simulink model "DoubleWishbone"  (Simulink 9.3)
settings: Solver=ode45  StartTime=0.0  StopTime=0.066  RelTol=1e-3  EnableMultiTasking=on
values from neighbouring files (symbols this model uses):
  s = solve(eqn,x)    [solver.m]
undefined symbols (not defined in the file): x
libraries: mblibv1 x47
settings Model: Creator=tdenery  LastModifiedBy=nicwiggins
settings DataIOCC: LimitDataPoints=on
settings OptimizationCC: InitFltsAndDblsToZero=on
settings DebuggingCC: SaveWithParameterizedLinksMsg=none  SignalResolutionControl=TryResolveAllWithWarning  MultiTaskDSMMsg=warning  MultiTaskCondExecSysMsg=none
settings HardwareCC: TargetBitPerLong=64  TargetBitPerPointer=64  TargetBitPerSizeT=64  TargetBitPerPtrDiffT=64  TargetLongLongMode=on  TargetIntDivRoundTo=Zero  TargetEndianess=LittleEndian  TargetWordSize=64  TargetHWDeviceType=MATLAB Host  ProdEqTarget=off
settings SFSimCC: SimUseLocalCustomCode=on
settings RTWCC: RTWUseLocalCustomCode=on
settings GRTTargetCC: TargetFcnLib=ansi_tfl_tmw.mat
settings ConfigComp: CovExternalEMLEnable=on

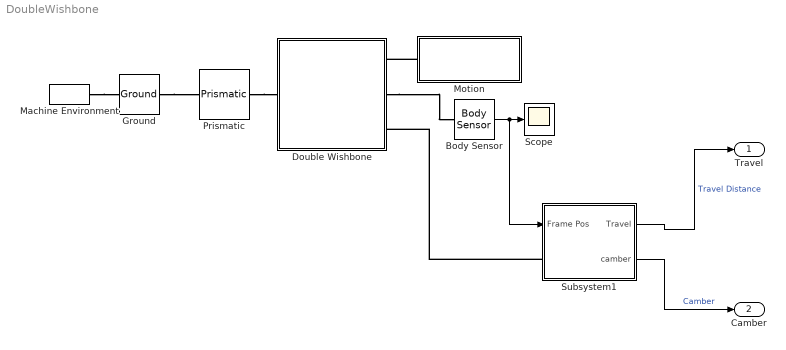
== system DoubleWishbone ==
  Body Sensor : mblibv1/Sensors &  Actuators/Body Sensor  UpdateFromCAD=off  PhysicalDomain=Mechanical  PortType=blob  Muxed=on  Pose=off  Angle=on  AngleUnits=deg  ArcVelocity=off  ArcVelocityUnits=deg/s  ArcAcceleration=off  ArcAccelerationUnits=deg/s^2  CoordPosition=on  CoordPositionUnits=m  Velocity=off  VelocityUnits=m/s  Acceleration=off  AccelerationUnits=m/s^2  Quaternion=on  QuaternionDT=off  QuaternionDDT=off  QuaternionUnits=off  OutputVector=[ 3 ]  ActiveIO=on  Width=3  DialogClass=MechanicalSensorBlock  ReferenceFrame=Absolute (World)
      settings: SourceProductName=Simscape Multibody  SourceProductBaseCode=MS
  Double Wishbone : Subsystem  mask(Double Wishbone Suspension){LU=x(1), UFPt=x(2:4), UBPt=x(5:7), LL=x(8), LFPt=x(9:11), LBPt=x(12:14), LC=x(15), k=300, b=20, Fps=20000}
      mask prompts: LU "Upper Arm Length (in)"; UFPt "Upper Arm Front Connection Point [x y z] (in)"; UBPt "Upper Arm Back Connection Point [x y z] (in)"; LL "Lower Arm Length (in)"; LFPt "Lower Arm Front Connection Point [x y z] (in)"; LBPt "Lower Arm Back Connection Point [x y z] (in)"; LC "Connecting Ling Length (in)"; k "Shock Spring Constant (lbf/in)"; b "Shock Damping Constant (lbf-s/in)"; Fps "Shock Pre-Set Force (lbf)"
      mask init:
      | UPV = UBPt - UFPt;
      | UBase = sqrt(UPV(1)^2+UPV(2)^2+UPV(3)^2);
      | ULink = sqrt(LU*LU + UBase*UBase/4);
      | LPV = LBPt - LFPt;
      | LBase = sqrt(LPV(1)^2+LPV(2)^2+LPV(3)^2);
      | LLink = sqrt(LL*LL + LBase*LBase/4);
  Ground : mblibv1/Bodies/Ground  UpdateFromCAD=off  LeftPortType=env  RightPortType=workingframe  PhysicalDomain=Mechanical  DialogClass=GroundBlock  CoordPosition=[0 0 0]  CoordPositionUnits=m  StateVectorMgrId=-1  MachineId=[0 0]  ShowEnvPort=on  ParameterChecksum=[0 0 0 0]  TopologyChecksum=[0 0 0 0]
      settings: SourceProductName=Simscape Multibody  SourceProductBaseCode=MS
  Machine Environment : mblibv1/Bodies/Machine Environment  Tag=Factory ground  PortType=env  PhysicalDomain=Mechanical  DialogTemplateClass=MECH.MachineEnvironment  SyncWhenCopied=off  Gravity=[0 -9.81 0]  GravityUnits=m/s^2  GravityAsSignal=off  Dimensionality=Auto-detect  AnalysisType=Forward dynamics  LinearAssemblyTolerance=1e-3  LinearAssemblyToleranceUnits=m  AngularAssemblyTolerance=1e-3  AngularAssemblyToleranceUnits=rad  ConstraintSolverType=Stabilizing  ConstraintRelTolerance=1e-4  ConstraintAbsTolerance=1e-4  UseRobustSingularityHandling=off  RedundancyAnalysisToleranceType=Automatically select tolerance  RedundancyAnalysisTolerance=1e-14  StatePerturbationType=Fixed  PerturbationSize=1e-5  VisualizeMachine=on  BodyVisualizationType=Use model default body geometries  BodyColorSelMode=Use model default  DefaultBodyColor=[1 0 0]
      settings: SourceProductName=Simscape Multibody  SourceProductBaseCode=MS
  Motion : Subsystem  mask{dhole=0.2, dtravel=30, speed=10}
      mask prompts: dhole "Pot Hole Depth (m)"; dtravel "Travel Distance to Hole (m)"; speed "Vehicle Speed (m/s)"
  Prismatic : mblibv1/Joints/Prismatic  LConnTagsString=__newl0  RConnTagsString=__newr0  UpdateFromCAD=off  NumSAPorts=0  CutJoint=off  MarkAsCut=off  Primitives=prismatic  PrimitiveProps=P1$WORLD$[0 1 0]$prismatic  DialogClass=JointBlock  P1Axis=[0 1 0]
      settings: SourceProductName=Simscape Multibody  SourceProductBaseCode=MS
  Scope : Scope
  Subsystem1 : Subsystem
  Travel : Outport
  Camber : Outport  Port=2
  wires:
  Body Sensor/1 -> Scope/1, Subsystem1/1(Frame Pos)
  Subsystem1/1(Travel) -> Travel/1  "Travel Distance"
  Subsystem1/2(camber) -> Camber/1  "Camber"
  connections:
  Machine Environment/RConn1 -- Ground/LConn1
  Ground/RConn1 -- Prismatic/LConn1
  Prismatic/RConn1 -- Double Wishbone/LConn1
  Motion/LConn1 -- Double Wishbone/RConn1
  Double Wishbone/RConn2 -- Body Sensor/LConn1
  Subsystem1/LConn1 -- Double Wishbone/RConn3

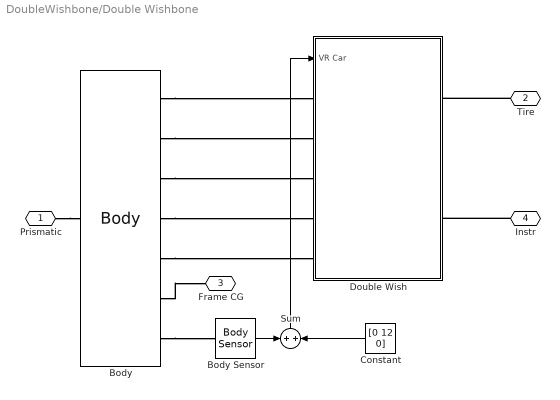
== system DoubleWishbone/Double Wishbone ==
  Body : mblibv1/Bodies/Body  LConnTagsString=CS1  RConnTagsString=CS2|CS3|CS4|CS5|CS6|CS7|CS8  UpdateFromCAD=off  DialogClass=MechanicalBodyBlock  Mass=1000  MassUnits=lbm  InertiaUnits=lbm*in^2  Inertia=eye(3)  Shape=Cylinder  ShapeDims=[1 1]  ShapeUnits=m  ShapeUse=false  Density=1  DensityUnits=kg/m^3  DensityUse=false  GraphicsMode=MACHINE_DEFAULT  BodyColorSelMode=MACHINE_DEFAULT  BodyColor=[1;0;0]  AttachedToCS=CG  CG=Left$CG$[0 0 0]$CS1$CS1$in$[0 0 0]$Euler X-Y-Z$deg$CS1$false  WorkingFrames=Left$CS1$[0 0 0]$ADJOINING$ADJOINING$in$[0 0 0]$Euler X-Y-Z$deg$ADJOINING$true#Right$CS2$UFPt$CG$CG$in$[0 0 0]$Euler X-Y-Z$deg$CG$true#Right$CS3$UBPt$CG$CG$in$[0 0 0]$Euler X-Y-Z$deg$CG$true#Right$CS4$LFPt$CG$CG$in$[0 0 0]$Euler X-Y-Z$deg$CG$true#Right$CS5$LBPt$CG$CG$in$[0 0 0]$Euler X-Y-Z$deg$CG$true#Right$CS6$[0 0 0]$ADJOINING$ADJOINING$in$[0 0 0]$Euler X-Y-Z$deg$ADJOINING$true#Right$CS7$[0 0 0]$CG$CG$in$[0 0 0]$Euler X-Y-Z$deg$WORLD$true#Right$CS8$[0 0 0]$CG$CG$m$[0 0 0]$Euler X-Y-Z$deg$CG$true  CGPos=[0 0 0]  CGRot=[0 0 0]  CS0Pos=[]  CS0Rot=[]  CS1Pos=[0 0 0]  CS1Rot=[0 0 0]  CS2Pos=UFPt  CS2Rot=[0 0 0]  CS3Pos=UBPt  CS3Rot=[0 0 0]  CS4Pos=LFPt  CS4Rot=[0 0 0]  CS5Pos=LBPt  CS5Rot=[0 0 0]  CS6Pos=[0 0 0]  CS6Rot=[0 0 0]  CS7Pos=[0 0 0]  CS7Rot=[0 0 0]  CS8Pos=[0 0 0]  CS8Rot=[0 0 0]  CS9Pos=[]  CS9Rot=[]  CS10Pos=[]  CS10Rot=[]  CS11Pos=[]  CS11Rot=[]  CS12Pos=[]  CS12Rot=[]  CS13Pos=[]  CS13Rot=[]  CS14Pos=[]  CS14Rot=[]  CS15Pos=[]  CS15Rot=[]  CS16Pos=[]  CS16Rot=[]  CS17Pos=[]  CS17Rot=[]  CS18Pos=[]  CS18Rot=[]  CS19Pos=[]  CS19Rot=[]  CS20Pos=[]  CS20Rot=[]
      settings: SourceProductName=Simscape Multibody  SourceProductBaseCode=MS
  Body Sensor : mblibv1/Sensors &  Actuators/Body Sensor  UpdateFromCAD=off  PhysicalDomain=Mechanical  PortType=blob  Muxed=on  Pose=off  Angle=on  AngleUnits=deg  ArcVelocity=off  ArcVelocityUnits=deg/s  ArcAcceleration=off  ArcAccelerationUnits=deg/s^2  CoordPosition=on  CoordPositionUnits=in  Velocity=off  VelocityUnits=m/s  Acceleration=off  AccelerationUnits=m/s^2  Quaternion=on  QuaternionDT=off  QuaternionDDT=off  QuaternionUnits=off  OutputVector=[ 3 ]  ActiveIO=on  Width=3  DialogClass=MechanicalSensorBlock  ReferenceFrame=Absolute (World)
      settings: SourceProductName=Simscape Multibody  SourceProductBaseCode=MS
  Constant : Constant  Value=[0 12 0]
  Double Wish : Subsystem
  Sum : Sum
  Prismatic : PMIOPort  Side=Left
  Tire : PMIOPort  Port=2  Side=Right
  Frame CG : PMIOPort  Port=3  Side=Right
  Instr : PMIOPort  Port=4  Side=Right
  wires:
  Body Sensor/1 -> Sum/1
  Constant/1 -> Sum/2
  Sum/1 -> Double Wish/1(VR Car)
  connections:
  Body/RConn1 -- Double Wish/LConn1
  Body/RConn2 -- Double Wish/LConn2
  Body/RConn3 -- Double Wish/LConn3
  Body/RConn4 -- Double Wish/LConn4
  Prismatic/RConn1 -- Body/LConn1
  Body/RConn5 -- Double Wish/LConn5
  Tire/RConn1 -- Double Wish/RConn1
  Body/RConn6 -- Frame CG/RConn1
  Instr/RConn1 -- Double Wish/RConn2
  Body/RConn7 -- Body Sensor/LConn1

== system DoubleWishbone/Motion ==
  Body : mblibv1/Bodies/Body  LConnTagsString=CS1  RConnTagsString=CS2  UpdateFromCAD=off  DialogClass=MechanicalBodyBlock  Mass=1  MassUnits=kg  InertiaUnits=kg*m^2  Inertia=eye(3)  Shape=Cylinder  ShapeDims=[1 1]  ShapeUnits=m  ShapeUse=false  Density=1  DensityUnits=kg/m^3  DensityUse=false  GraphicsMode=MACHINE_DEFAULT  BodyColorSelMode=MACHINE_DEFAULT  BodyColor=[1;0;0]  AttachedToCS=CG  CG=Left$CG$[0 0 0]$CS2$CS2$m$[0 0 0]$Euler X-Y-Z$deg$CS2$false  WorkingFrames=Left$CS1$[0 0 0]$CG$CG$m$[0 0 0]$Euler X-Y-Z$deg$CG$true#Right$CS2$[0 0 0]$ADJOINING$ADJOINING$m$[0 0 0]$Euler X-Y-Z$deg$ADJOINING$true  CGPos=[0 0 0]  CGRot=[0 0 0]  CS0Pos=[]  CS0Rot=[]  CS1Pos=[0 0 0]  CS1Rot=[0 0 0]  CS2Pos=[0 0 0]  CS2Rot=[0 0 0]  CS3Pos=[]  CS3Rot=[]  CS4Pos=[]  CS4Rot=[]  CS5Pos=[]  CS5Rot=[]  CS6Pos=[]  CS6Rot=[]  CS7Pos=[]  CS7Rot=[]  CS8Pos=[]  CS8Rot=[]  CS9Pos=[]  CS9Rot=[]  CS10Pos=[]  CS10Rot=[]  CS11Pos=[]  CS11Rot=[]  CS12Pos=[]  CS12Rot=[]  CS13Pos=[]  CS13Rot=[]  CS14Pos=[]  CS14Rot=[]  CS15Pos=[]  CS15Rot=[]  CS16Pos=[]  CS16Rot=[]  CS17Pos=[]  CS17Rot=[]  CS18Pos=[]  CS18Rot=[]  CS19Pos=[]  CS19Rot=[]  CS20Pos=[]  CS20Rot=[]
      settings: SourceProductName=Simscape Multibody  SourceProductBaseCode=MS
  Gaussian Pulse Position : Subsystem  mask{magnitude=-dhole, sigma=1, distance=dtravel, speed=speed}
      mask prompts: magnitude "Peak Value"; sigma "Standard Deviation"; distance "Distance to Bump (m)"; speed "Vehicle Speed (m/s)"
  Ground : mblibv1/Bodies/Ground  UpdateFromCAD=off  LeftPortType=env  RightPortType=workingframe  PhysicalDomain=Mechanical  DialogClass=GroundBlock  CoordPosition=[0 0 0]  CoordPositionUnits=m  StateVectorMgrId=-1  MachineId=[0 0]  ShowEnvPort=off  ParameterChecksum=[0 0 0 0]  TopologyChecksum=[0 0 0 0]
      settings: SourceProductName=Simscape Multibody  SourceProductBaseCode=MS
  Joint Actuator : mblibv1/Sensors &  Actuators/Joint Actuator  UpdateFromCAD=off  PhysicalDomain=Mechanical  PortType=blob  ActuationStyle=Motion  AngleUnits=deg  ArcVelocityUnits=deg/s  ArcAccelerationUnits=deg/s^2  CoordPositionUnits=m  VelocityUnits=m/s  AccelerationUnits=m/s^2  ForceUnits=N  TorqueUnits=N-m  ActiveIO=on  Width=3  DialogClass=MechanicalActuatorBlock  Primitive=P2  ReferenceFrame=Absolute (INERTIAL)
      settings: SourceProductName=Simscape Multibody  SourceProductBaseCode=MS
  Six-DoF : mblibv1/Joints/Six-DoF  LConnTagsString=__newl0|SA1  RConnTagsString=__newr0  UpdateFromCAD=off  NumSAPorts=1  CutJoint=off  MarkAsCut=off  Primitives=prismatic_prismatic_prismatic_spherical  PrimitiveProps=P1$WORLD$[1 0 0]$prismatic#P2$WORLD$[0 1 0]$prismatic#P3$WORLD$[0 0 1]$prismatic#S$WORLD$[0 0 0]$spherical  DialogClass=JointBlock  P1Axis=[1 0 0]  P2Axis=[0 1 0]  P3Axis=[0 0 1]  SAxis=[0 0 0]
      settings: SourceProductName=Simscape Multibody  SourceProductBaseCode=MS
  Weld : mblibv1/Joints/Weld  LConnTagsString=__newl0  RConnTagsString=__newr0  UpdateFromCAD=off  NumSAPorts=0  CutJoint=off  MarkAsCut=off  Primitives=weld  PrimitiveProps=W$INERTIAL$[0 0 0]$weld  DialogClass=JointBlock  WAxis=[0 0 0]
      settings: SourceProductName=Simscape Multibody  SourceProductBaseCode=MS
  Motion : PMIOPort  Tag=PMCPort  Side=Left
  wires:
  Gaussian Pulse Position/1(PVA) -> Joint Actuator/1
  connections:
  Ground/RConn1 -- Six-DoF/LConn1
  Joint Actuator/RConn1 -- Six-DoF/LConn2
  Weld/RConn1 -- Motion/RConn1
  Six-DoF/RConn1 -- Body/LConn1
  Body/RConn1 -- Weld/LConn1

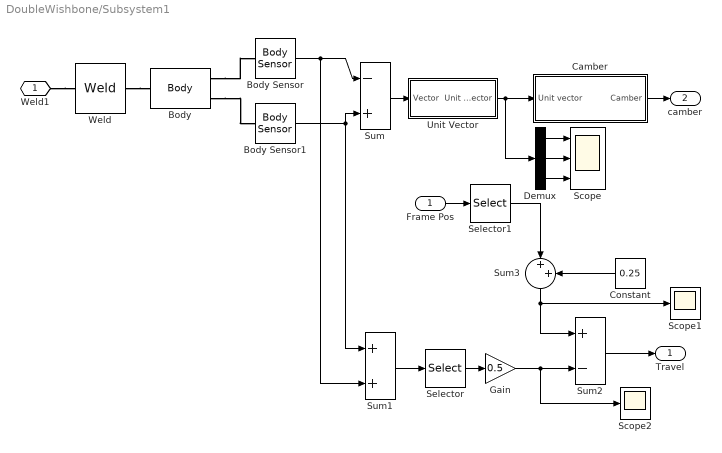
== system DoubleWishbone/Subsystem1 ==
  Frame Pos : Inport
  Body : mblibv1/Bodies/Body  LConnTagsString=CG  RConnTagsString=CS1|CS2  UpdateFromCAD=off  DialogClass=MechanicalBodyBlock  Mass=1  MassUnits=kg  InertiaUnits=kg*m^2  Inertia=eye(3)  Shape=Cylinder  ShapeDims=[1 1]  ShapeUnits=m  ShapeUse=false  Density=1  DensityUnits=kg/m^3  DensityUse=false  GraphicsMode=MACHINE_DEFAULT  BodyColorSelMode=MACHINE_DEFAULT  BodyColor=[1;0;0]  AttachedToCS=CG  CG=Left$CG$[0 0 0]$ADJOINING$ADJOINING$in$[0 0 0]$Euler X-Y-Z$deg$ADJOINING$true  WorkingFrames=Right$CS1$[0 1 0]$CG$CG$in$[0 0 0]$Euler X-Y-Z$deg$CG$true#Right$CS2$[0 -1 0]$CG$CG$in$[0 0 0]$Euler X-Y-Z$deg$CG$true  CGPos=[0 0 0]  CGRot=[0 0 0]  CS0Pos=[]  CS0Rot=[]  CS1Pos=[0 1 0]  CS1Rot=[0 0 0]  CS2Pos=[0 -1 0]  CS2Rot=[0 0 0]  CS3Pos=[]  CS3Rot=[]  CS4Pos=[]  CS4Rot=[]  CS5Pos=[]  CS5Rot=[]  CS6Pos=[]  CS6Rot=[]  CS7Pos=[]  CS7Rot=[]  CS8Pos=[]  CS8Rot=[]  CS9Pos=[]  CS9Rot=[]  CS10Pos=[]  CS10Rot=[]  CS11Pos=[]  CS11Rot=[]  CS12Pos=[]  CS12Rot=[]  CS13Pos=[]  CS13Rot=[]  CS14Pos=[]  CS14Rot=[]  CS15Pos=[]  CS15Rot=[]  CS16Pos=[]  CS16Rot=[]  CS17Pos=[]  CS17Rot=[]  CS18Pos=[]  CS18Rot=[]  CS19Pos=[]  CS19Rot=[]  CS20Pos=[]  CS20Rot=[]
      settings: SourceProductName=Simscape Multibody  SourceProductBaseCode=MS
  Body Sensor : mblibv1/Sensors &  Actuators/Body Sensor  UpdateFromCAD=off  PhysicalDomain=Mechanical  PortType=blob  Muxed=on  Pose=off  Angle=on  AngleUnits=deg  ArcVelocity=off  ArcVelocityUnits=deg/s  ArcAcceleration=off  ArcAccelerationUnits=deg/s^2  CoordPosition=on  CoordPositionUnits=m  Velocity=off  VelocityUnits=m/s  Acceleration=off  AccelerationUnits=m/s^2  Quaternion=on  QuaternionDT=off  QuaternionDDT=off  QuaternionUnits=off  OutputVector=[ 3 ]  ActiveIO=on  Width=3  DialogClass=MechanicalSensorBlock  ReferenceFrame=Absolute (World)
      settings: SourceProductName=Simscape Multibody  SourceProductBaseCode=MS
  Body Sensor1 : mblibv1/Sensors &  Actuators/Body Sensor  UpdateFromCAD=off  PhysicalDomain=Mechanical  PortType=blob  Muxed=on  Pose=off  Angle=on  AngleUnits=deg  ArcVelocity=off  ArcVelocityUnits=deg/s  ArcAcceleration=off  ArcAccelerationUnits=deg/s^2  CoordPosition=on  CoordPositionUnits=m  Velocity=off  VelocityUnits=m/s  Acceleration=off  AccelerationUnits=m/s^2  Quaternion=on  QuaternionDT=off  QuaternionDDT=off  QuaternionUnits=off  OutputVector=[ 3 ]  ActiveIO=on  Width=3  DialogClass=MechanicalSensorBlock  ReferenceFrame=Absolute (World)
      settings: SourceProductName=Simscape Multibody  SourceProductBaseCode=MS
  Camber : Subsystem
  Constant : Constant  Value=0.25
  Demux : Demux  Outputs=3
  Gain : Gain  Gain=0.5
  Scope : Scope  NumInputPorts=3
  Scope1 : Scope
  Scope2 : Scope
  Selector : Selector  InputPortWidth=3  IndexOptions=Index vector (dialog)  Indices=[2]  OutputSizes=1
  Selector1 : Selector  InputPortWidth=3  IndexOptions=Index vector (dialog)  Indices=[2]  OutputSizes=1
  Sum : Sum  Inputs=-+
  Sum1 : Sum
  Sum2 : Sum  Inputs=+-
  Sum3 : Sum  Inputs=|++
  Unit Vector : Subsystem
  Weld : mblibv1/Joints/Weld  LConnTagsString=__newl0  RConnTagsString=__newr0  UpdateFromCAD=off  NumSAPorts=0  CutJoint=off  MarkAsCut=off  Primitives=weld  PrimitiveProps=W$INERTIAL$[0 0 0]$weld  DialogClass=JointBlock  WAxis=[0 0 0]
      settings: SourceProductName=Simscape Multibody  SourceProductBaseCode=MS
  Weld1 : PMIOPort  Side=Left
  Travel : Outport
  camber : Outport  Port=2
  wires:
  Body Sensor/1 -> Sum/1, Sum1/2
  Body Sensor1/1 -> Sum/2, Sum1/1
  Camber/1(Camber) -> camber/1
  Sum/1 -> Unit Vector/1(Vector)
  Unit Vector/1(Unit Vector) -> Camber/1(Unit vector), Demux/1
  Demux/1 -> Scope/1
  Demux/2 -> Scope/2
  Demux/3 -> Scope/3
  Selector/1 -> Gain/1
  Sum1/1 -> Selector/1
  Frame Pos/1 -> Selector1/1
  Gain/1 -> Sum2/2, Scope2/1
  Sum2/1 -> Travel/1
  Selector1/1 -> Sum3/1
  Sum3/1 -> Sum2/1, Scope1/1
  Constant/1 -> Sum3/2
  connections:
  Weld1/RConn1 -- Weld/LConn1
  Weld/RConn1 -- Body/LConn1
  Body/RConn1 -- Body Sensor/LConn1
  Body/RConn2 -- Body Sensor1/LConn1

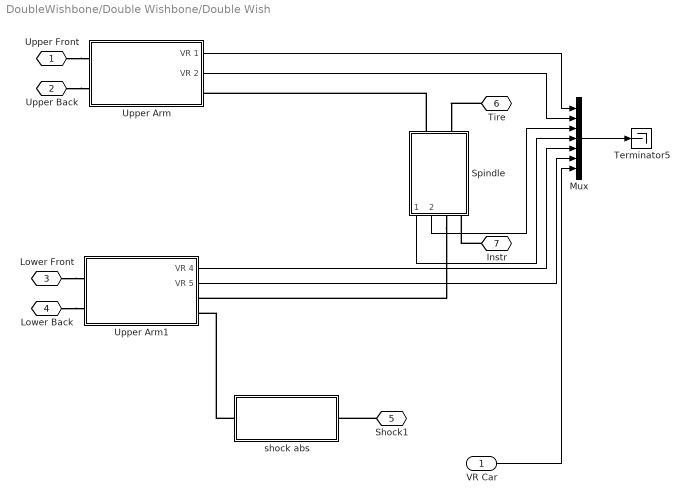
== system DoubleWishbone/Double Wishbone/Double Wish ==
  VR Car : Inport
  Mux : Mux  Inputs=7
  Spindle : Subsystem  mask{r=0.25, h=12, rho=0.05, Rot=[0 0 -90]}
      mask prompts: r "Radius (in)"; h "Height (in)"; rho "Material Density (lbm/in^3)"; Rot "Rotation [Rx, Ry, Rz] (degrees)"
  Terminator5 : Terminator
  Upper Arm : Subsystem
  Upper Arm1 : Subsystem
  shock abs : Subsystem
  Upper Front : PMIOPort  Side=Left
  Upper Back : PMIOPort  Port=2  Side=Left
  Lower Front : PMIOPort  Port=3  Side=Left
  Lower Back : PMIOPort  Port=4  Side=Left
  Shock1 : PMIOPort  Port=5  Side=Left
  "Tire " : PMIOPort  Port=6  Side=Right
  Instr : PMIOPort  Port=7  Side=Right
  wires:
  Upper Arm/1(VR 1) -> Mux/1
  Upper Arm/2(VR 2) -> Mux/2
  Spindle/2(VR 6) -> Mux/3
  Spindle/1(VR 3) -> Mux/4
  Upper Arm1/1(VR 4) -> Mux/5
  Upper Arm1/2(VR 5) -> Mux/6
  VR Car/1 -> Mux/7
  Mux/1 -> Terminator5/1
  connections:
  "Tire "/RConn1 -- Spindle/LConn2
  Instr/RConn1 -- Spindle/RConn2
  shock abs/LConn1 -- Upper Arm1/RConn2
  Shock1/RConn1 -- shock abs/RConn1
  Lower Back/RConn1 -- Upper Arm1/LConn2
  Lower Front/RConn1 -- Upper Arm1/LConn1
  Upper Back/RConn1 -- Upper Arm/LConn2
  Upper Front/RConn1 -- Upper Arm/LConn1
  Spindle/LConn1 -- Upper Arm/RConn1
  Spindle/RConn1 -- Upper Arm1/RConn1

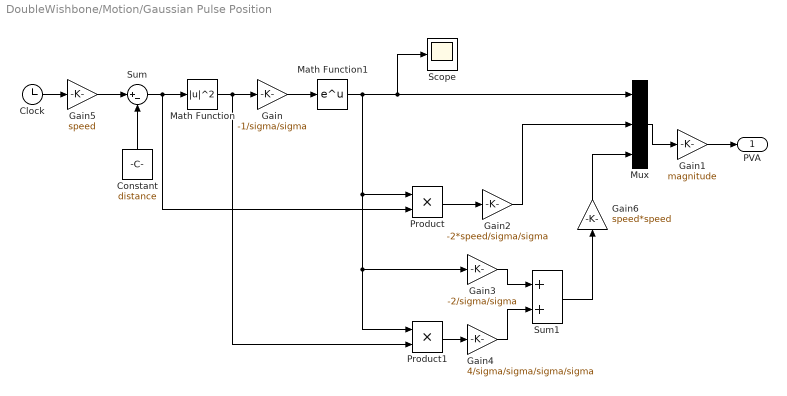
== system DoubleWishbone/Motion/Gaussian Pulse Position ==
  Clock : Clock
  Constant : Constant  Value=distance
  Gain : Gain  Gain=-1/sigma/sigma
  Gain1 : Gain  Gain=magnitude
  Gain2 : Gain  Gain=-2*speed/sigma/sigma
  Gain3 : Gain  Gain=-2/sigma/sigma
  Gain4 : Gain  Gain=4/sigma/sigma/sigma/sigma
  Gain5 : Gain  Gain=speed
  Gain6 : Gain  Gain=speed*speed
  Math Function : Math  Operator=magnitude^2  SaturateOnIntegerOverflow=on
  Math Function1 : Math  SaturateOnIntegerOverflow=on
  Mux : Mux  Inputs=3
  Product : Product  RndMeth=Zero
  Product1 : Product  RndMeth=Zero
  Scope : Scope
  Sum : Sum  Inputs=|+-
  Sum1 : Sum
  PVA : Outport
  wires:
  Constant/1 -> Sum/2
  Sum/1 -> Math Function/1, Product/2
  Math Function/1 -> Gain/1, Product1/2
  Gain/1 -> Math Function1/1
  Math Function1/1 -> Product/1, Product1/1, Gain3/1, Mux/1, Scope/1
  Product/1 -> Gain2/1
  Gain2/1 -> Mux/2
  Mux/1 -> Gain1/1
  Gain1/1 -> PVA/1
  Product1/1 -> Gain4/1
  Gain3/1 -> Sum1/1
  Gain4/1 -> Sum1/2
  Sum1/1 -> Gain6/1
  Clock/1 -> Gain5/1
  Gain5/1 -> Sum/1
  Gain6/1 -> Mux/3

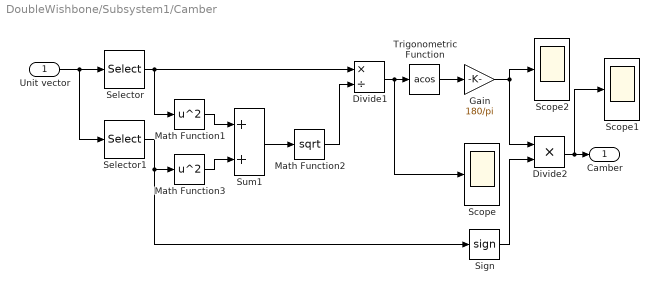
== system DoubleWishbone/Subsystem1/Camber ==
  Unit vector : Inport
  Divide1 : Product  Inputs=*/
  Divide2 : Product  Inputs=**
  Gain : Gain  Gain=180/pi
  Math Function1 : Math  Operator=square  SaturateOnIntegerOverflow=on
  Math Function2 : Math  Operator=sqrt  SaturateOnIntegerOverflow=on
  Math Function3 : Math  Operator=square  SaturateOnIntegerOverflow=on
  Scope : Scope
  Scope1 : Scope
  Scope2 : Scope
  Selector : Selector  InputPortWidth=3  IndexOptions=Index vector (dialog)  Indices=2  OutputSizes=1
  Selector1 : Selector  InputPortWidth=3  IndexOptions=Index vector (dialog)  Indices=1  OutputSizes=1
  Sign : Signum  ZeroCross=off
  Sum1 : Sum
  Trigonometric Function : Trigonometry  Operator=acos
  Camber : Outport
  wires:
  Unit vector/1 -> Selector1/1, Selector/1
  Selector/1 -> Divide1/1, Math Function1/1
  Selector1/1 -> Math Function3/1, Sign/1
  Math Function1/1 -> Sum1/1
  Math Function3/1 -> Sum1/2
  Sum1/1 -> Math Function2/1
  Math Function2/1 -> Divide1/2
  Divide1/1 -> Trigonometric Function/1, Scope/1
  Trigonometric Function/1 -> Gain/1
  Gain/1 -> Divide2/1, Scope2/1
  Sign/1 -> Divide2/2
  Divide2/1 -> Camber/1, Scope1/1

== system DoubleWishbone/Subsystem1/Unit Vector ==
  Vector : Inport
  Divide : Product  Inputs=*/
  Dot Product : DotProduct  InputSameDT=on  OutDataTypeStr=Inherit: Inherit via internal rule
  Math Function : Math  Operator=sqrt  SaturateOnIntegerOverflow=on
  Unit Vector : Outport
  wires:
  Vector/1 -> Dot Product/2, Dot Product/1, Divide/1
  Dot Product/1 -> Math Function/1
  Math Function/1 -> Divide/2
  Divide/1 -> Unit Vector/1

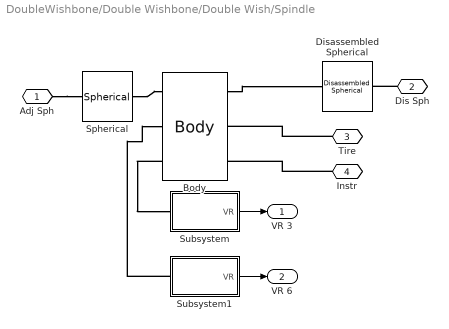
== system DoubleWishbone/Double Wishbone/Double Wish/Spindle ==
  Body : mblibv1/Bodies/Body  LConnTagsString=CS1|CS5|CG  RConnTagsString=CS2|CS3|CS4  UpdateFromCAD=off  DialogClass=MechanicalBodyBlock  Mass=rho*pi*r*r*h  MassUnits=lbm  InertiaUnits=lbm*in^2  Inertia=rho*pi*r*r*h*[(3*r*r + h*h) 0 0;0 6*r*r 0;0 0 (3*r*r + h*h)]/12  Shape=Cylinder  ShapeDims=[1 1]  ShapeUnits=m  ShapeUse=false  Density=1  DensityUnits=kg/m^3  DensityUse=false  GraphicsMode=MACHINE_DEFAULT  BodyColorSelMode=MACHINE_DEFAULT  BodyColor=[1;0;0]  AttachedToCS=CG  CG=Left$CG$[0 h/2 0]$CS1$CS1$in$[0 0 0]$Euler X-Y-Z$deg$CS1$true  WorkingFrames=Left$CS1$[0 0 0]$ADJOINING$ADJOINING$in$Rot$Euler X-Y-Z$deg$ADJOINING$true#Right$CS2$[0 h/2 0]$CG$CG$in$[0 0 0]$Euler X-Y-Z$deg$CG$true#Right$CS3$[0 0 0]$CG$CG$m$[0 0 0]$Euler X-Y-Z$deg$WORLD$true#Right$CS4$[0 0 0]$CG$CG$m$[0 0 0]$Euler X-Y-Z$deg$CG$true#Left$CS5$[0 0 0]$CG$CG$m$[0 0 115]$Euler X-Y-Z$deg$CG$true  CGPos=[0 h/2 0]  CGRot=[0 0 0]  CS0Pos=[]  CS0Rot=[]  CS1Pos=[0 0 0]  CS1Rot=Rot  CS2Pos=[0 h/2 0]  CS2Rot=[0 0 0]  CS3Pos=[0 0 0]  CS3Rot=[0 0 0]  CS4Pos=[0 0 0]  CS4Rot=[0 0 0]  CS5Pos=[0 0 0]  CS5Rot=[0 0 115]  CS6Pos=[]  CS6Rot=[]  CS7Pos=[]  CS7Rot=[]  CS8Pos=[]  CS8Rot=[]  CS9Pos=[]  CS9Rot=[]  CS10Pos=[]  CS10Rot=[]  CS11Pos=[]  CS11Rot=[]  CS12Pos=[]  CS12Rot=[]  CS13Pos=[]  CS13Rot=[]  CS14Pos=[]  CS14Rot=[]  CS15Pos=[]  CS15Rot=[]  CS16Pos=[]  CS16Rot=[]  CS17Pos=[]  CS17Rot=[]  CS18Pos=[]  CS18Rot=[]  CS19Pos=[]  CS19Rot=[]  CS20Pos=[]  CS20Rot=[]
      settings: SourceProductName=Simscape Multibody  SourceProductBaseCode=MS
  Disassembled Spherical : mblibv1/Joints/Disassembled Joints/Disassembled Spherical  LConnTagsString=__newl0  RConnTagsString=__newr0  UpdateFromCAD=off  DialogClass=JointBlock  Primitives=prismatic_prismatic  PrimitiveProps=Base$INERTIAL$[1 0 0]$prismatic#Follower$INERTIAL$[0 1 0]$prismatic  BaseAxis=[1 0 0]  FollowerAxis=[0 1 0]
      settings: SourceProductName=Simscape Multibody  SourceProductBaseCode=MS
  Spherical : mblibv1/Joints/Spherical  LConnTagsString=__newl0  RConnTagsString=__newr0  UpdateFromCAD=off  NumSAPorts=0  CutJoint=off  MarkAsCut=off  Primitives=spherical  PrimitiveProps=S$INERTIAL$[0 0 0]$spherical  DialogClass=JointBlock  SAxis=[0 0 0]
      settings: SourceProductName=Simscape Multibody  SourceProductBaseCode=MS
  Subsystem : Subsystem
  Subsystem1 : Subsystem
  Adj Sph : PMIOPort  Side=Left
  Dis Sph : PMIOPort  Port=2  Side=Right
  Tire : PMIOPort  Port=3  Side=Left
  Instr : PMIOPort  Port=4  Side=Right
  VR 3 : Outport
  VR 6 : Outport  Port=2
  wires:
  Subsystem/1(VR) -> VR 3/1
  Subsystem1/1(VR) -> VR 6/1
  connections:
  Instr/RConn1 -- Body/RConn3
  Tire/RConn1 -- Body/RConn2
  Body/LConn3 -- Subsystem/LConn1
  Spherical/RConn1 -- Body/LConn1
  Adj Sph/RConn1 -- Spherical/LConn1
  Dis Sph/RConn1 -- Disassembled Spherical/RConn1
  Body/RConn1 -- Disassembled Spherical/LConn1
  Subsystem1/LConn1 -- Body/LConn2

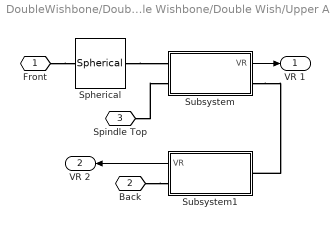
== system DoubleWishbone/Double Wishbone/Double Wish/Upper Arm ==
  Spherical : mblibv1/Joints/Spherical  LConnTagsString=__newl0  RConnTagsString=__newr0  UpdateFromCAD=off  NumSAPorts=0  CutJoint=off  MarkAsCut=off  Primitives=spherical  PrimitiveProps=S$INERTIAL$[0 0 0]$spherical  DialogClass=JointBlock  SAxis=[0 0 0]
      settings: SourceProductName=Simscape Multibody  SourceProductBaseCode=MS
  Subsystem : Subsystem  mask{r=0.25, h=ULink, rho=0.05, Rot=[0 0 -90]}
      mask prompts: r "Radius (in)"; h "Height (in)"; rho "Material Density (lbm/in^3)"; Rot "Rotation [Rx, Ry, Rz] (degrees)"
  Subsystem1 : Subsystem  mask{r=0.25, h=ULink, rho=0.05, Rot=[-150 0 0]}
      mask prompts: r "Radius (in)"; h "Height (in)"; rho "Material Density (lbm/in^3)"; Rot "Rotation [Rx, Ry, Rz] (degrees)"
  Front : PMIOPort  Side=Left
  Back : PMIOPort  Port=2  Side=Left
  Spindle Top : PMIOPort  Port=3  Side=Right
  VR 1 : Outport
  VR 2 : Outport  Port=2
  wires:
  Subsystem1/1(VR) -> VR 2/1
  Subsystem/1(VR) -> VR 1/1
  connections:
  Spindle Top/RConn1 -- Subsystem/LConn2
  Back/RConn1 -- Subsystem1/RConn1
  Front/RConn1 -- Spherical/LConn1
  Subsystem/RConn1 -- Subsystem1/LConn1
  Spherical/RConn1 -- Subsystem/LConn1

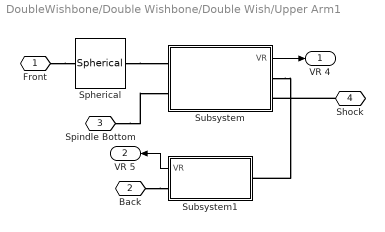
== system DoubleWishbone/Double Wishbone/Double Wish/Upper Arm1 ==
  Spherical : mblibv1/Joints/Spherical  LConnTagsString=__newl0  RConnTagsString=__newr0  UpdateFromCAD=off  NumSAPorts=0  CutJoint=off  MarkAsCut=off  Primitives=spherical  PrimitiveProps=S$INERTIAL$[0 0 0]$spherical  DialogClass=JointBlock  SAxis=[0 0 0]
      settings: SourceProductName=Simscape Multibody  SourceProductBaseCode=MS
  Subsystem : Subsystem  mask{r=0.25, h=LLink, rho=0.05, Rot=[0 0 -90]}
      mask prompts: r "Radius (in)"; h "Height (in)"; rho "Material Density (lbm/in^3)"; Rot "Rotation [Rx, Ry, Rz] (degrees)"
  Subsystem1 : Subsystem  mask{r=0.25, h=LLink, rho=0.05, Rot=[130 0 0]}
      mask prompts: r "Radius (in)"; h "Height (in)"; rho "Material Density (lbm/in^3)"; Rot "Rotation [Rx, Ry, Rz] (degrees)"
  Front : PMIOPort  Side=Left
  Back : PMIOPort  Port=2  Side=Left
  Spindle Bottom : PMIOPort  Port=3  Side=Right
  Shock : PMIOPort  Port=4  Side=Right
  VR 4 : Outport
  VR 5 : Outport  Port=2
  wires:
  Subsystem1/1(VR) -> VR 5/1
  Subsystem/1(VR) -> VR 4/1
  connections:
  Shock/RConn1 -- Subsystem/RConn2
  Spindle Bottom/RConn1 -- Subsystem/LConn2
  Back/RConn1 -- Subsystem1/RConn1
  Front/RConn1 -- Spherical/LConn1
  Spherical/RConn1 -- Subsystem/LConn1
  Subsystem/RConn1 -- Subsystem1/LConn1

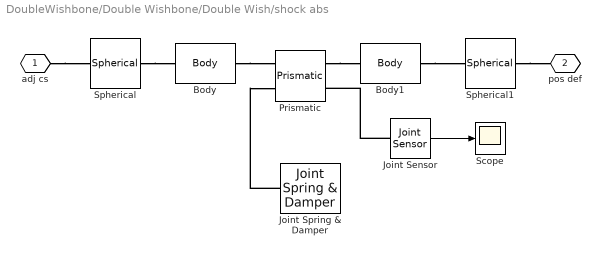
== system DoubleWishbone/Double Wishbone/Double Wish/shock abs ==
  Body : mblibv1/Bodies/Body  LConnTagsString=CS1  RConnTagsString=CS2  UpdateFromCAD=off  DialogClass=MechanicalBodyBlock  Mass=1  MassUnits=kg  InertiaUnits=kg*m^2  Inertia=eye(3)  Shape=Cylinder  ShapeDims=[1 1]  ShapeUnits=m  ShapeUse=false  Density=1  DensityUnits=kg/m^3  DensityUse=false  GraphicsMode=MACHINE_DEFAULT  BodyColorSelMode=MACHINE_DEFAULT  BodyColor=[1;0;0]  AttachedToCS=CG  CG=Left$CG$[0 0 0]$CS1$CS1$in$[0 0 0]$Euler X-Y-Z$deg$CS1$false  WorkingFrames=Left$CS1$[0 0 0]$ADJOINING$ADJOINING$in$[0 0 0]$Euler X-Y-Z$deg$WORLD$true#Right$CS2$[0 0 0]$CG$CG$in$[0 0 0]$Euler X-Y-Z$deg$CG$true  CGPos=[0 0 0]  CGRot=[0 0 0]  CS0Pos=[]  CS0Rot=[]  CS1Pos=[0 0 0]  CS1Rot=[0 0 0]  CS2Pos=[0 0 0]  CS2Rot=[0 0 0]  CS3Pos=[]  CS3Rot=[]  CS4Pos=[]  CS4Rot=[]  CS5Pos=[]  CS5Rot=[]  CS6Pos=[]  CS6Rot=[]  CS7Pos=[]  CS7Rot=[]  CS8Pos=[]  CS8Rot=[]  CS9Pos=[]  CS9Rot=[]  CS10Pos=[]  CS10Rot=[]  CS11Pos=[]  CS11Rot=[]  CS12Pos=[]  CS12Rot=[]  CS13Pos=[]  CS13Rot=[]  CS14Pos=[]  CS14Rot=[]  CS15Pos=[]  CS15Rot=[]  CS16Pos=[]  CS16Rot=[]  CS17Pos=[]  CS17Rot=[]  CS18Pos=[]  CS18Rot=[]  CS19Pos=[]  CS19Rot=[]  CS20Pos=[]  CS20Rot=[]
      settings: SourceProductName=Simscape Multibody  SourceProductBaseCode=MS
  Body1 : mblibv1/Bodies/Body  LConnTagsString=CS1  RConnTagsString=CS2  UpdateFromCAD=off  DialogClass=MechanicalBodyBlock  Mass=1  MassUnits=kg  InertiaUnits=kg*m^2  Inertia=eye(3)  Shape=Cylinder  ShapeDims=[1 1]  ShapeUnits=m  ShapeUse=false  Density=1  DensityUnits=kg/m^3  DensityUse=false  GraphicsMode=MACHINE_DEFAULT  BodyColorSelMode=MACHINE_DEFAULT  BodyColor=[1;0;0]  AttachedToCS=CG  CG=Left$CG$[0 0 0]$CS1$CS1$in$[0 0 0]$Euler X-Y-Z$deg$CS1$false  WorkingFrames=Left$CS1$[0 20 0]$ADJOINING$ADJOINING$in$[0 0 0]$Euler X-Y-Z$deg$ADJOINING$true#Right$CS2$[0 0 0]$CG$CG$in$[0 0 0]$Euler X-Y-Z$deg$CG$true  CGPos=[0 0 0]  CGRot=[0 0 0]  CS0Pos=[]  CS0Rot=[]  CS1Pos=[0 20 0]  CS1Rot=[0 0 0]  CS2Pos=[0 0 0]  CS2Rot=[0 0 0]  CS3Pos=[]  CS3Rot=[]  CS4Pos=[]  CS4Rot=[]  CS5Pos=[]  CS5Rot=[]  CS6Pos=[]  CS6Rot=[]  CS7Pos=[]  CS7Rot=[]  CS8Pos=[]  CS8Rot=[]  CS9Pos=[]  CS9Rot=[]  CS10Pos=[]  CS10Rot=[]  CS11Pos=[]  CS11Rot=[]  CS12Pos=[]  CS12Rot=[]  CS13Pos=[]  CS13Rot=[]  CS14Pos=[]  CS14Rot=[]  CS15Pos=[]  CS15Rot=[]  CS16Pos=[]  CS16Rot=[]  CS17Pos=[]  CS17Rot=[]  CS18Pos=[]  CS18Rot=[]  CS19Pos=[]  CS19Rot=[]  CS20Pos=[]  CS20Rot=[]
      settings: SourceProductName=Simscape Multibody  SourceProductBaseCode=MS
  Joint Sensor : mblibv1/Sensors &  Actuators/Joint Sensor  UpdateFromCAD=off  PhysicalDomain=Mechanical  PortType=blob  Muxed=on  Pose=off  Angle=on  AngleUnits=deg  ArcVelocity=off  ArcVelocityUnits=deg/s  ArcAcceleration=off  ArcAccelerationUnits=deg/s^2  CoordPosition=off  CoordPositionUnits=m  Velocity=off  VelocityUnits=m/s  Acceleration=off  AccelerationUnits=m/s^2  Quaternion=on  QuaternionDT=off  QuaternionDDT=off  QuaternionUnits=off  OutputVector=[ 1 ]  ActiveIO=on  Width=1  DialogClass=MechanicalSensorBlock  Primitive=P1  Force=on  ForceUnits=lb  Torque=off  TorqueUnits=N-m  ReferenceFrame=Absolute (INERTIAL)  ReactionSensedSide=Base  ReactionReferenceFrame=Absolute (World)  ReactionForce=off  ReactionForceUnits=N  ReactionMoment=off  ReactionMomentUnits=N-m
      settings: SourceProductName=Simscape Multibody  SourceProductBaseCode=MS
  Joint Spring & Damper : mblibv1/Force  Elements/Joint Spring & Damper  UpdateFromCAD=off  DialogClass=JointSpringDamper  JFEParameters=P1$true$k$b$Fps/k$in$in/s$lb$rad$rad/s$N-m#P2$false$0$0$0$m$m/s$N$rad$rad/s$N-m#P3$false$0$0$0$m$m/s$N$rad$rad/s$N-m#R1$false$0$0$0$m$m/s$N$rad$rad/s$N-m#R2$false$0$0$0$m$m/s$N$rad$rad/s$N-m#R3$false$0$0$0$m$m/s$N$rad$rad/s$N-m#S$false$0$0$0$m$m/s$N$rad$rad/s$N-m
      settings: SourceProductName=Simscape Multibody  SourceProductBaseCode=MS
  Prismatic : mblibv1/Joints/Prismatic  LConnTagsString=__newl0|SA1  RConnTagsString=__newr0|SA1  UpdateFromCAD=off  NumSAPorts=2  CutJoint=off  MarkAsCut=off  Primitives=prismatic  PrimitiveProps=P1$Base$[0 1 0]$prismatic  DialogClass=JointBlock  P1Axis=[0 1 0]
      settings: SourceProductName=Simscape Multibody  SourceProductBaseCode=MS
  Scope : Scope
  Spherical : mblibv1/Joints/Spherical  LConnTagsString=__newl0  RConnTagsString=__newr0  UpdateFromCAD=off  NumSAPorts=0  CutJoint=off  MarkAsCut=off  Primitives=spherical  PrimitiveProps=S$INERTIAL$[0 0 0]$spherical  DialogClass=JointBlock  SAxis=[0 0 0]
      settings: SourceProductName=Simscape Multibody  SourceProductBaseCode=MS
  Spherical1 : mblibv1/Joints/Spherical  LConnTagsString=__newl0  RConnTagsString=__newr0  UpdateFromCAD=off  NumSAPorts=0  CutJoint=off  MarkAsCut=off  Primitives=spherical  PrimitiveProps=S$INERTIAL$[0 0 0]$spherical  DialogClass=JointBlock  SAxis=[0 0 0]
      settings: SourceProductName=Simscape Multibody  SourceProductBaseCode=MS
  adj cs : PMIOPort  Tag=PMCPort  Side=Left
  pos def : PMIOPort  Tag=PMCPort  Port=2  Side=Right
  wires:
  Joint Sensor/1 -> Scope/1
  connections:
  Joint Spring & Damper/LConn1 -- Prismatic/LConn2
  Body/RConn1 -- Prismatic/LConn1
  adj cs/RConn1 -- Spherical/LConn1
  Spherical/RConn1 -- Body/LConn1
  Prismatic/RConn1 -- Body1/LConn1
  Body1/RConn1 -- Spherical1/LConn1
  Spherical1/RConn1 -- pos def/RConn1
  Joint Sensor/LConn1 -- Prismatic/RConn2

== system DoubleWishbone/Double Wishbone/Double Wish/Spindle/Subsystem ==
  Body Sensor : mblibv1/Sensors &  Actuators/Body Sensor  UpdateFromCAD=off  PhysicalDomain=Mechanical  PortType=blob  Muxed=off  Pose=on  Angle=on  AngleUnits=deg  ArcVelocity=off  ArcVelocityUnits=deg/s  ArcAcceleration=off  ArcAccelerationUnits=deg/s^2  CoordPosition=on  CoordPositionUnits=in  Velocity=off  VelocityUnits=m/s  Acceleration=off  AccelerationUnits=m/s^2  Quaternion=on  QuaternionDT=off  QuaternionDDT=off  QuaternionUnits=off  OutputVector=[ 3 9 ]  ActiveIO=on  Width=12  DialogClass=MechanicalSensorBlock  ReferenceFrame=Absolute (World)
      settings: SourceProductName=Simscape Multibody  SourceProductBaseCode=MS
  Bus Creator : BusCreator  Inputs=4
  Convert from Rotation Matrix to Virtual Reality Toolbox : mblibv1/Utilities/Convert from Rotation Matrix to Simulink 3D Animation format  Tag=Pose2VR
      settings: SourceProductName=Simscape Multibody  SourceProductBaseCode=MS
  Height : Constant  Value=h
  Radius : Constant  Value=r
  CG : PMIOPort  Side=Left
  VR : Outport
  wires:
  Bus Creator/1 -> VR/1
  Radius/1 -> Bus Creator/4  "Radius"
  Height/1 -> Bus Creator/3  "Height"
  Convert from Rotation Matrix to Virtual Reality Toolbox/1 -> Bus Creator/2  "Rotation"
  Body Sensor/1 -> Bus Creator/1  "Translation"
  Body Sensor/2 -> Convert from Rotation Matrix to Virtual Reality Toolbox/1
  connections:
  CG/RConn1 -- Body Sensor/LConn1

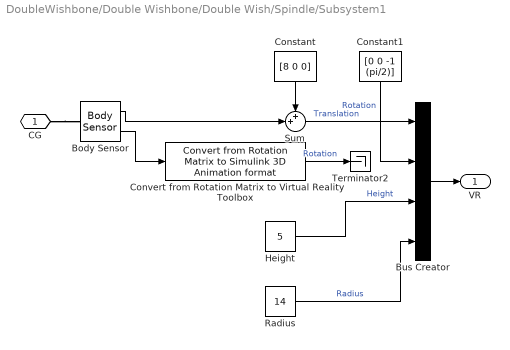
== system DoubleWishbone/Double Wishbone/Double Wish/Spindle/Subsystem1 ==
  Body Sensor : mblibv1/Sensors &  Actuators/Body Sensor  UpdateFromCAD=off  PhysicalDomain=Mechanical  PortType=blob  Muxed=off  Pose=on  Angle=on  AngleUnits=deg  ArcVelocity=off  ArcVelocityUnits=deg/s  ArcAcceleration=off  ArcAccelerationUnits=deg/s^2  CoordPosition=on  CoordPositionUnits=in  Velocity=off  VelocityUnits=m/s  Acceleration=off  AccelerationUnits=m/s^2  Quaternion=on  QuaternionDT=off  QuaternionDDT=off  QuaternionUnits=off  OutputVector=[ 3 9 ]  ActiveIO=on  Width=12  DialogClass=MechanicalSensorBlock  ReferenceFrame=Absolute (World)
      settings: SourceProductName=Simscape Multibody  SourceProductBaseCode=MS
  Bus Creator : BusCreator  Inputs=4
  Constant : Constant  Value=[8 0 0]
  Constant1 : Constant  Value=[0 0 -1 (pi/2)]
  Convert from Rotation Matrix to Virtual Reality Toolbox : mblibv1/Utilities/Convert from Rotation Matrix to Simulink 3D Animation format  Tag=Pose2VR
      settings: SourceProductName=Simscape Multibody  SourceProductBaseCode=MS
  Height : Constant  Value=5
  Radius : Constant  Value=14
  Sum : Sum  Inputs=++|
  Terminator2 : Terminator
  CG : PMIOPort  Side=Left
  VR : Outport
  wires:
  Height/1 -> Bus Creator/3  "Height"
  Radius/1 -> Bus Creator/4  "Radius"
  Bus Creator/1 -> VR/1
  Constant/1 -> Sum/1
  Body Sensor/1 -> Sum/2
  Sum/1 -> Bus Creator/1  "Translation"
  Body Sensor/2 -> Convert from Rotation Matrix to Virtual Reality Toolbox/1
  Constant1/1 -> Bus Creator/2  "Rotation"
  Convert from Rotation Matrix to Virtual Reality Toolbox/1 -> Terminator2/1  "Rotation"
  connections:
  CG/RConn1 -- Body Sensor/LConn1

== system DoubleWishbone/Double Wishbone/Double Wish/Upper Arm/Subsystem ==
  Body : mblibv1/Bodies/Body  LConnTagsString=CS1|CG  RConnTagsString=CS2|CS3  UpdateFromCAD=off  DialogClass=MechanicalBodyBlock  Mass=rho*pi*r*r*h  MassUnits=lbm  InertiaUnits=lbm*in^2  Inertia=rho*pi*r*r*h*[(3*r*r + h*h) 0 0;0 6*r*r 0;0 0 (3*r*r + h*h)]/12  Shape=Cylinder  ShapeDims=[1 1]  ShapeUnits=m  ShapeUse=false  Density=1  DensityUnits=kg/m^3  DensityUse=false  GraphicsMode=MACHINE_DEFAULT  BodyColorSelMode=MACHINE_DEFAULT  BodyColor=[1;0;0]  AttachedToCS=CG  CG=Left$CG$[0 h/2 0]$CS1$CS1$in$[0 0 0]$Euler X-Y-Z$deg$CS1$true  WorkingFrames=Left$CS1$[0 0 0]$ADJOINING$ADJOINING$in$Rot$Euler X-Y-Z$deg$ADJOINING$true#Right$CS2$[0 h/2 0]$CG$CG$in$[0 0 0]$Euler X-Y-Z$deg$CG$true#Right$CS3$[0 0 0]$CS2$CS2$m$[0 0 0]$Euler X-Y-Z$deg$CS2$true  CGPos=[0 h/2 0]  CGRot=[0 0 0]  CS0Pos=[]  CS0Rot=[]  CS1Pos=[0 0 0]  CS1Rot=Rot  CS2Pos=[0 h/2 0]  CS2Rot=[0 0 0]  CS3Pos=[0 0 0]  CS3Rot=[0 0 0]  CS4Pos=[]  CS4Rot=[]  CS5Pos=[]  CS5Rot=[]  CS6Pos=[]  CS6Rot=[]  CS7Pos=[]  CS7Rot=[]  CS8Pos=[]  CS8Rot=[]  CS9Pos=[]  CS9Rot=[]  CS10Pos=[]  CS10Rot=[]  CS11Pos=[]  CS11Rot=[]  CS12Pos=[]  CS12Rot=[]  CS13Pos=[]  CS13Rot=[]  CS14Pos=[]  CS14Rot=[]  CS15Pos=[]  CS15Rot=[]  CS16Pos=[]  CS16Rot=[]  CS17Pos=[]  CS17Rot=[]  CS18Pos=[]  CS18Rot=[]  CS19Pos=[]  CS19Rot=[]  CS20Pos=[]  CS20Rot=[]
      settings: SourceProductName=Simscape Multibody  SourceProductBaseCode=MS
  Revolute : mblibv1/Joints/Revolute  LConnTagsString=__newl0  RConnTagsString=__newr0  UpdateFromCAD=off  NumSAPorts=0  CutJoint=off  MarkAsCut=off  Primitives=revolute  PrimitiveProps=R1$Base$[1 0 0]$revolute  DialogClass=JointBlock  R1Axis=[1 0 0]
      settings: SourceProductName=Simscape Multibody  SourceProductBaseCode=MS
  Subsystem : Subsystem
  Adj CS : PMIOPort  Side=Left
  Rev : PMIOPort  Port=2  Side=Right
  Spindle Top : PMIOPort  Port=3  Side=Left
  VR : Outport
  wires:
  Subsystem/1(VR) -> VR/1
  connections:
  Subsystem/LConn1 -- Body/LConn2
  Body/RConn2 -- Spindle Top/RConn1
  Rev/RConn1 -- Revolute/RConn1
  Adj CS/RConn1 -- Body/LConn1
  Body/RConn1 -- Revolute/LConn1

== system DoubleWishbone/Double Wishbone/Double Wish/Upper Arm/Subsystem1 ==
  Body : mblibv1/Bodies/Body  LConnTagsString=CS1|CG  RConnTagsString=CS2  UpdateFromCAD=off  DialogClass=MechanicalBodyBlock  Mass=rho*pi*r*r*h  MassUnits=lbm  InertiaUnits=lbm*in^2  Inertia=rho*pi*r*r*h*[(3*r*r + h*h) 0 0;0 6*r*r 0;0 0 (3*r*r + h*h)]/12  Shape=Cylinder  ShapeDims=[1 1]  ShapeUnits=m  ShapeUse=false  Density=1  DensityUnits=kg/m^3  DensityUse=false  GraphicsMode=MACHINE_DEFAULT  BodyColorSelMode=MACHINE_DEFAULT  BodyColor=[1;0;0]  AttachedToCS=CG  CG=Left$CG$[0 h/2 0]$CS1$CS1$in$[0 0 0]$Euler X-Y-Z$deg$CS1$true  WorkingFrames=Left$CS1$[0 0 0]$ADJOINING$ADJOINING$in$Rot$Euler X-Y-Z$deg$ADJOINING$true#Right$CS2$[0 h/2 0]$CG$CG$in$[0 0 0]$Euler X-Y-Z$deg$CG$true  CGPos=[0 h/2 0]  CGRot=[0 0 0]  CS0Pos=[]  CS0Rot=[]  CS1Pos=[0 0 0]  CS1Rot=Rot  CS2Pos=[0 h/2 0]  CS2Rot=[0 0 0]  CS3Pos=[]  CS3Rot=[]  CS4Pos=[]  CS4Rot=[]  CS5Pos=[]  CS5Rot=[]  CS6Pos=[]  CS6Rot=[]  CS7Pos=[]  CS7Rot=[]  CS8Pos=[]  CS8Rot=[]  CS9Pos=[]  CS9Rot=[]  CS10Pos=[]  CS10Rot=[]  CS11Pos=[]  CS11Rot=[]  CS12Pos=[]  CS12Rot=[]  CS13Pos=[]  CS13Rot=[]  CS14Pos=[]  CS14Rot=[]  CS15Pos=[]  CS15Rot=[]  CS16Pos=[]  CS16Rot=[]  CS17Pos=[]  CS17Rot=[]  CS18Pos=[]  CS18Rot=[]  CS19Pos=[]  CS19Rot=[]  CS20Pos=[]  CS20Rot=[]
      settings: SourceProductName=Simscape Multibody  SourceProductBaseCode=MS
  Disassembled Spherical : mblibv1/Joints/Disassembled Joints/Disassembled Spherical  LConnTagsString=__newl0  RConnTagsString=__newr0  UpdateFromCAD=off  DialogClass=JointBlock  Primitives=prismatic_prismatic  PrimitiveProps=Base$INERTIAL$[1 0 0]$prismatic#Follower$INERTIAL$[0 1 0]$prismatic  BaseAxis=[1 0 0]  FollowerAxis=[0 1 0]
      settings: SourceProductName=Simscape Multibody  SourceProductBaseCode=MS
  Subsystem : Subsystem
  Adj CS : PMIOPort  Side=Left
  Dis Sph : PMIOPort  Port=2  Side=Right
  VR : Outport
  wires:
  Subsystem/1(VR) -> VR/1
  connections:
  Subsystem/LConn1 -- Body/LConn2
  Body/RConn1 -- Disassembled Spherical/LConn1
  Adj CS/RConn1 -- Body/LConn1
  Dis Sph/RConn1 -- Disassembled Spherical/RConn1

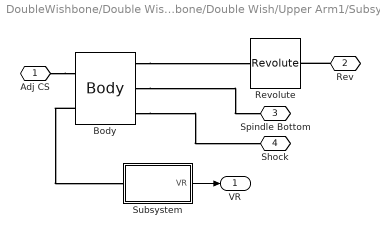
== system DoubleWishbone/Double Wishbone/Double Wish/Upper Arm1/Subsystem ==
  Body : mblibv1/Bodies/Body  LConnTagsString=CS1|CG  RConnTagsString=CS2|CS3|CS4  UpdateFromCAD=off  DialogClass=MechanicalBodyBlock  Mass=rho*pi*r*r*h  MassUnits=lbm  InertiaUnits=lbm*in^2  Inertia=rho*pi*r*r*h*[(3*r*r + h*h) 0 0;0 6*r*r 0;0 0 (3*r*r + h*h)]/12  Shape=Cylinder  ShapeDims=[1 1]  ShapeUnits=m  ShapeUse=false  Density=1  DensityUnits=kg/m^3  DensityUse=false  GraphicsMode=MACHINE_DEFAULT  BodyColorSelMode=MACHINE_DEFAULT  BodyColor=[1;0;0]  AttachedToCS=CG  CG=Left$CG$[0 h/2 0]$CS1$CS1$in$[0 0 0]$Euler X-Y-Z$deg$CS1$true  WorkingFrames=Left$CS1$[0 0 0]$ADJOINING$ADJOINING$in$Rot$Euler X-Y-Z$deg$ADJOINING$true#Right$CS2$[0 h/2 0]$CG$CG$in$[0 0 0]$Euler X-Y-Z$deg$CG$true#Right$CS3$[0 0 0]$CS2$CS2$in$[0 0 0]$Euler X-Y-Z$deg$CS2$true#Right$CS4$[0 h/6 -h/12]$CG$CG$in$[0 0 0]$Euler X-Y-Z$deg$WORLD$true  CGPos=[0 h/2 0]  CGRot=[0 0 0]  CS0Pos=[]  CS0Rot=[]  CS1Pos=[0 0 0]  CS1Rot=Rot  CS2Pos=[0 h/2 0]  CS2Rot=[0 0 0]  CS3Pos=[0 0 0]  CS3Rot=[0 0 0]  CS4Pos=[0 h/6 -h/12]  CS4Rot=[0 0 0]  CS5Pos=[]  CS5Rot=[]  CS6Pos=[]  CS6Rot=[]  CS7Pos=[]  CS7Rot=[]  CS8Pos=[]  CS8Rot=[]  CS9Pos=[]  CS9Rot=[]  CS10Pos=[]  CS10Rot=[]  CS11Pos=[]  CS11Rot=[]  CS12Pos=[]  CS12Rot=[]  CS13Pos=[]  CS13Rot=[]  CS14Pos=[]  CS14Rot=[]  CS15Pos=[]  CS15Rot=[]  CS16Pos=[]  CS16Rot=[]  CS17Pos=[]  CS17Rot=[]  CS18Pos=[]  CS18Rot=[]  CS19Pos=[]  CS19Rot=[]  CS20Pos=[]  CS20Rot=[]
      settings: SourceProductName=Simscape Multibody  SourceProductBaseCode=MS
  Revolute : mblibv1/Joints/Revolute  LConnTagsString=__newl0  RConnTagsString=__newr0  UpdateFromCAD=off  NumSAPorts=0  CutJoint=off  MarkAsCut=off  Primitives=revolute  PrimitiveProps=R1$Base$[1 0 0]$revolute  DialogClass=JointBlock  R1Axis=[1 0 0]
      settings: SourceProductName=Simscape Multibody  SourceProductBaseCode=MS
  Subsystem : Subsystem
  Adj CS : PMIOPort  Side=Left
  Rev : PMIOPort  Port=2  Side=Right
  Spindle Bottom : PMIOPort  Port=3  Side=Left
  Shock : PMIOPort  Port=4  Side=Right
  VR : Outport
  wires:
  Subsystem/1(VR) -> VR/1
  connections:
  Body/RConn3 -- Shock/RConn1
  Body/LConn2 -- Subsystem/LConn1
  Body/RConn2 -- Spindle Bottom/RConn1
  Rev/RConn1 -- Revolute/RConn1
  Adj CS/RConn1 -- Body/LConn1
  Body/RConn1 -- Revolute/LConn1

== system DoubleWishbone/Double Wishbone/Double Wish/Upper Arm1/Subsystem1 ==
  Body : mblibv1/Bodies/Body  LConnTagsString=CS1|CG  RConnTagsString=CS2  UpdateFromCAD=off  DialogClass=MechanicalBodyBlock  Mass=rho*pi*r*r*h  MassUnits=lbm  InertiaUnits=lbm*in^2  Inertia=rho*pi*r*r*h*[(3*r*r + h*h) 0 0;0 6*r*r 0;0 0 (3*r*r + h*h)]/12  Shape=Cylinder  ShapeDims=[1 1]  ShapeUnits=m  ShapeUse=false  Density=1  DensityUnits=kg/m^3  DensityUse=false  GraphicsMode=MACHINE_DEFAULT  BodyColorSelMode=MACHINE_DEFAULT  BodyColor=[1;0;0]  AttachedToCS=CG  CG=Left$CG$[0 h/2 0]$CS1$CS1$in$[0 0 0]$Euler X-Y-Z$deg$CS1$true  WorkingFrames=Left$CS1$[0 0 0]$ADJOINING$ADJOINING$in$Rot$Euler X-Y-Z$deg$ADJOINING$true#Right$CS2$[0 h/2 0]$CG$CG$in$[0 0 0]$Euler X-Y-Z$deg$CG$true  CGPos=[0 h/2 0]  CGRot=[0 0 0]  CS0Pos=[]  CS0Rot=[]  CS1Pos=[0 0 0]  CS1Rot=Rot  CS2Pos=[0 h/2 0]  CS2Rot=[0 0 0]  CS3Pos=[]  CS3Rot=[]  CS4Pos=[]  CS4Rot=[]  CS5Pos=[]  CS5Rot=[]  CS6Pos=[]  CS6Rot=[]  CS7Pos=[]  CS7Rot=[]  CS8Pos=[]  CS8Rot=[]  CS9Pos=[]  CS9Rot=[]  CS10Pos=[]  CS10Rot=[]  CS11Pos=[]  CS11Rot=[]  CS12Pos=[]  CS12Rot=[]  CS13Pos=[]  CS13Rot=[]  CS14Pos=[]  CS14Rot=[]  CS15Pos=[]  CS15Rot=[]  CS16Pos=[]  CS16Rot=[]  CS17Pos=[]  CS17Rot=[]  CS18Pos=[]  CS18Rot=[]  CS19Pos=[]  CS19Rot=[]  CS20Pos=[]  CS20Rot=[]
      settings: SourceProductName=Simscape Multibody  SourceProductBaseCode=MS
  Disassembled Spherical : mblibv1/Joints/Disassembled Joints/Disassembled Spherical  LConnTagsString=__newl0  RConnTagsString=__newr0  UpdateFromCAD=off  DialogClass=JointBlock  Primitives=prismatic_prismatic  PrimitiveProps=Base$INERTIAL$[1 0 0]$prismatic#Follower$INERTIAL$[0 1 0]$prismatic  BaseAxis=[1 0 0]  FollowerAxis=[0 1 0]
      settings: SourceProductName=Simscape Multibody  SourceProductBaseCode=MS
  Subsystem : Subsystem
  Adj CS : PMIOPort  Side=Left
  Dis Sph : PMIOPort  Port=2  Side=Right
  VR : Outport
  wires:
  Subsystem/1(VR) -> VR/1
  connections:
  Subsystem/LConn1 -- Body/LConn2
  Body/RConn1 -- Disassembled Spherical/LConn1
  Adj CS/RConn1 -- Body/LConn1
  Dis Sph/RConn1 -- Disassembled Spherical/RConn1

== system DoubleWishbone/Double Wishbone/Double Wish/Upper Arm/Subsystem/Subsystem ==
  Body Sensor : mblibv1/Sensors &  Actuators/Body Sensor  UpdateFromCAD=off  PhysicalDomain=Mechanical  PortType=blob  Muxed=off  Pose=on  Angle=on  AngleUnits=deg  ArcVelocity=off  ArcVelocityUnits=deg/s  ArcAcceleration=off  ArcAccelerationUnits=deg/s^2  CoordPosition=on  CoordPositionUnits=in  Velocity=off  VelocityUnits=m/s  Acceleration=off  AccelerationUnits=m/s^2  Quaternion=on  QuaternionDT=off  QuaternionDDT=off  QuaternionUnits=off  OutputVector=[ 3 9 ]  ActiveIO=on  Width=12  DialogClass=MechanicalSensorBlock  ReferenceFrame=Absolute (World)
      settings: SourceProductName=Simscape Multibody  SourceProductBaseCode=MS
  Bus Creator : BusCreator  Inputs=4
  Convert from Rotation Matrix to Virtual Reality Toolbox : mblibv1/Utilities/Convert from Rotation Matrix to Simulink 3D Animation format  Tag=Pose2VR
      settings: SourceProductName=Simscape Multibody  SourceProductBaseCode=MS
  Height : Constant  Value=h
  Radius : Constant  Value=r
  CG : PMIOPort  Side=Left
  VR : Outport
  wires:
  Bus Creator/1 -> VR/1
  Radius/1 -> Bus Creator/4  "Radius"
  Height/1 -> Bus Creator/3  "Height"
  Convert from Rotation Matrix to Virtual Reality Toolbox/1 -> Bus Creator/2  "Rotation"
  Body Sensor/1 -> Bus Creator/1  "Translation"
  Body Sensor/2 -> Convert from Rotation Matrix to Virtual Reality Toolbox/1
  connections:
  CG/RConn1 -- Body Sensor/LConn1

== system DoubleWishbone/Double Wishbone/Double Wish/Upper Arm/Subsystem1/Subsystem ==
  Body Sensor : mblibv1/Sensors &  Actuators/Body Sensor  UpdateFromCAD=off  PhysicalDomain=Mechanical  PortType=blob  Muxed=off  Pose=on  Angle=on  AngleUnits=deg  ArcVelocity=off  ArcVelocityUnits=deg/s  ArcAcceleration=off  ArcAccelerationUnits=deg/s^2  CoordPosition=on  CoordPositionUnits=in  Velocity=off  VelocityUnits=m/s  Acceleration=off  AccelerationUnits=m/s^2  Quaternion=on  QuaternionDT=off  QuaternionDDT=off  QuaternionUnits=off  OutputVector=[ 3 9 ]  ActiveIO=on  Width=12  DialogClass=MechanicalSensorBlock  ReferenceFrame=Absolute (World)
      settings: SourceProductName=Simscape Multibody  SourceProductBaseCode=MS
  Bus Creator : BusCreator  Inputs=4
  Convert from Rotation Matrix to Virtual Reality Toolbox : mblibv1/Utilities/Convert from Rotation Matrix to Simulink 3D Animation format  Tag=Pose2VR
      settings: SourceProductName=Simscape Multibody  SourceProductBaseCode=MS
  Height : Constant  Value=h
  Radius : Constant  Value=r
  CG : PMIOPort  Side=Left
  VR : Outport
  wires:
  Bus Creator/1 -> VR/1
  Radius/1 -> Bus Creator/4  "Radius"
  Height/1 -> Bus Creator/3  "Height"
  Convert from Rotation Matrix to Virtual Reality Toolbox/1 -> Bus Creator/2  "Rotation"
  Body Sensor/1 -> Bus Creator/1  "Translation"
  Body Sensor/2 -> Convert from Rotation Matrix to Virtual Reality Toolbox/1
  connections:
  CG/RConn1 -- Body Sensor/LConn1

== system DoubleWishbone/Double Wishbone/Double Wish/Upper Arm1/Subsystem/Subsystem ==
  Body Sensor : mblibv1/Sensors &  Actuators/Body Sensor  UpdateFromCAD=off  PhysicalDomain=Mechanical  PortType=blob  Muxed=off  Pose=on  Angle=on  AngleUnits=deg  ArcVelocity=off  ArcVelocityUnits=deg/s  ArcAcceleration=off  ArcAccelerationUnits=deg/s^2  CoordPosition=on  CoordPositionUnits=in  Velocity=off  VelocityUnits=m/s  Acceleration=off  AccelerationUnits=m/s^2  Quaternion=on  QuaternionDT=off  QuaternionDDT=off  QuaternionUnits=off  OutputVector=[ 3 9 ]  ActiveIO=on  Width=12  DialogClass=MechanicalSensorBlock  ReferenceFrame=Absolute (World)
      settings: SourceProductName=Simscape Multibody  SourceProductBaseCode=MS
  Bus Creator : BusCreator  Inputs=4
  Convert from Rotation Matrix to Virtual Reality Toolbox : mblibv1/Utilities/Convert from Rotation Matrix to Simulink 3D Animation format  Tag=Pose2VR
      settings: SourceProductName=Simscape Multibody  SourceProductBaseCode=MS
  Height : Constant  Value=h
  Radius : Constant  Value=r
  CG : PMIOPort  Side=Left
  VR : Outport
  wires:
  Bus Creator/1 -> VR/1
  Radius/1 -> Bus Creator/4  "Radius"
  Height/1 -> Bus Creator/3  "Height"
  Convert from Rotation Matrix to Virtual Reality Toolbox/1 -> Bus Creator/2  "Rotation"
  Body Sensor/1 -> Bus Creator/1  "Translation"
  Body Sensor/2 -> Convert from Rotation Matrix to Virtual Reality Toolbox/1
  connections:
  CG/RConn1 -- Body Sensor/LConn1

== system DoubleWishbone/Double Wishbone/Double Wish/Upper Arm1/Subsystem1/Subsystem ==
  Body Sensor : mblibv1/Sensors &  Actuators/Body Sensor  UpdateFromCAD=off  PhysicalDomain=Mechanical  PortType=blob  Muxed=off  Pose=on  Angle=on  AngleUnits=deg  ArcVelocity=off  ArcVelocityUnits=deg/s  ArcAcceleration=off  ArcAccelerationUnits=deg/s^2  CoordPosition=on  CoordPositionUnits=in  Velocity=off  VelocityUnits=m/s  Acceleration=off  AccelerationUnits=m/s^2  Quaternion=on  QuaternionDT=off  QuaternionDDT=off  QuaternionUnits=off  OutputVector=[ 3 9 ]  ActiveIO=on  Width=12  DialogClass=MechanicalSensorBlock  ReferenceFrame=Absolute (World)
      settings: SourceProductName=Simscape Multibody  SourceProductBaseCode=MS
  Bus Creator : BusCreator  Inputs=4
  Convert from Rotation Matrix to Virtual Reality Toolbox : mblibv1/Utilities/Convert from Rotation Matrix to Simulink 3D Animation format  Tag=Pose2VR
      settings: SourceProductName=Simscape Multibody  SourceProductBaseCode=MS
  Height : Constant  Value=h
  Radius : Constant  Value=r
  CG : PMIOPort  Side=Left
  VR : Outport
  wires:
  Bus Creator/1 -> VR/1
  Radius/1 -> Bus Creator/4  "Radius"
  Height/1 -> Bus Creator/3  "Height"
  Convert from Rotation Matrix to Virtual Reality Toolbox/1 -> Bus Creator/2  "Rotation"
  Body Sensor/1 -> Bus Creator/1  "Translation"
  Body Sensor/2 -> Convert from Rotation Matrix to Virtual Reality Toolbox/1
  connections:
  CG/RConn1 -- Body Sensor/LConn1
